simulink model "bumpem_control_system"  (R2021b)
settings: Solver=ode4  StartTime=0.0  StopTime=Inf  FixedStep=0.001  RelTol=1e-3
PostLoadFcn:
  | , if any(exist('dsrtsu_mdlpostloadfcn', 'file') == [2, 3, 6]), try dsrtsu_mdlpostloadfcn('Execute', bdroot); catch fprintf('Error in PostLoadFcn (dsrtsu_mdlpostloadfcn) for model "%s":\n %s\n', bdroot, lasterr); end, end,
libraries: rti1202lib_dac_class1 x4, simulink x4, dsparch4 x2, rti1202lib_adc_class1 x2
(part 1 of 2)
PreSaveFcn:
  | , if any(exist('dsmpb_private', 'file') == [2, 3, 6]), try, dsmpb_private('dsmpb_mdlclblib', 'PreSave', bdroot); catch, disp(lasterr); end, end,
CloseFcn:
  | , if any(exist('dsmpb_private', 'file') == [2, 3, 6]), try, dsmpb_private('dsmpb_mdlclblib', 'Close', bdroot); catch, disp(lasterr); end, end,
Description:
  | Standard RTI1202 template.
  | Supported MATLAB version:  R2018a.
settings Model: Tag=RTI1202  DSRTSU_INTERNAL_RTI_VER=520  DSRTSU_INTERNAL_RTI_TYPE=rti1202  RTICANMMDATA=struct('GeneralSetupData',struct('modelroot',['C:\Users\HuMoTech\Documents\Bump Em\simulink'],'generalsettings',struct('filesettings',struct('destfolder',struct('Name','RTICANMM_FILES','Check',1),'buildfolder',struct('Name','.','Check',1),'AbsDestfolder',struct('Name',['C:\Users\HuMoTech\Documents\Bump Em\simulink\RTICANMM_FILES']),'AbsBuildfolder',struct('Name',['C:\Users\HuMoTech\Documents\Bump Em\simulink']))),'options',struct('addpaths',1,'rmpaths',1,'addtrcexclusion',logical(1),'cannavigator',struct('checkmonitoring',0),'show_usrtrc',0,'use_usrtrc',0),'advanced',struct('options',[1 1 1 1 1 1 1 1 1 1 1 1 1 1 1 1 1 1 1 1 1 1 1 1 1 1 1 1 1 1 1 1 1 1 1 1 1 1 1 1 1 1 1 1 1 1 1 1 1 1 1 1 1 1 1 1 1 1 1 1 1 1 1 1 1 1 1 1 1 1 1 1 1 1 1 1 1 1 1 1 1 1 1 1 1 1 1 1 1 1 1 1 1 1 1 1 1 1 1 1]),'MPSetup',{{}},'modelname','latest_version_control_system_v2','block','latest_version_control_system_v2'))  DSRTSU_INTERNAL_RTIFLEXRAYCONFIG=110  DSRTSU_INTERNAL_RTIFPGA=110  DSMPB_DATASERVER_ModelPortLibVersion1=8  DSMPB_DATASERVER_DataServerVersion1=6  DSMPB_DATASERVER_DataServerStreamVersion1=3  Creator=HuMoTech  LastModifiedBy=maxia
settings SolverCC: AlgebraicLoopSolver=TrustRegion
settings DataIOCC: ReturnWorkspaceOutputs=off
settings OptimizationCC: BlockReduction=off  OptimizeBlockIOStorage=off  BufferReuse=off  GlobalBufferReuse=off  ExpressionFolding=off  LocalBlockOutputs=off  OptimizeDataStoreBuffers=off  BusAssignmentInplaceUpdate=off
settings DebuggingCC: SFMachineParentedDataDiag=warning  ArithmeticOperatorsInVariantConditions=warning
settings HardwareCC: ProdBitPerPointer=32  ProdBitPerSizeT=32  ProdBitPerPtrDiffT=32  ProdLargestAtomicInteger=Integer  ProdEndianess=BigEndian  ProdWordSize=32  ProdHWDeviceType=Custom Processor->Custom  TargetIntDivRoundTo=Zero  TargetEndianess=BigEndian  TargetHWDeviceType=Custom Processor->Custom
settings SFSimCC: SimUseLocalCustomCode=off  MATLABDynamicMemAlloc=off  CustomCodeUndefinedFunction=UseInterfaceOnly
settings RTWCC: Description=dSPACE DS1202 Hardware Platform  SystemTargetFile=rti1202.tlc  MakeCommand=make_rti  TemplateMakefile=rti1202.tmf  RTWUseLocalCustomCode=off
settings CodeAppCC: StateflowObjectComments=on
settings STFCustomTargetCC: ParMdlRefBuildCompliant=on  GRTInterface=off  SystemTargetFile=rti1202.tlc
settings GRTTargetCC: TargetLangStandard=C89/C90 (ANSI)  CompOptLevelCompliant=off  ConcurrentExecutionCompliant=off  CombineOutputUpdateFcns=off  MatFileLogging=off  CPPClassGenCompliant=off  UseToolchainInfoCompliant=off
settings ConfigComp: CovMetricSettings=dswe

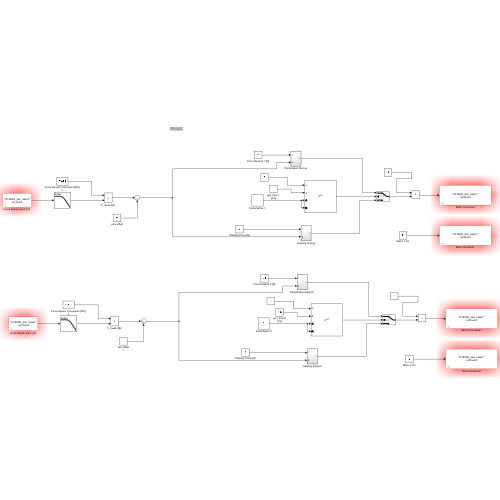
[thumbnail: Simulink's stored preview of the top-level diagram]
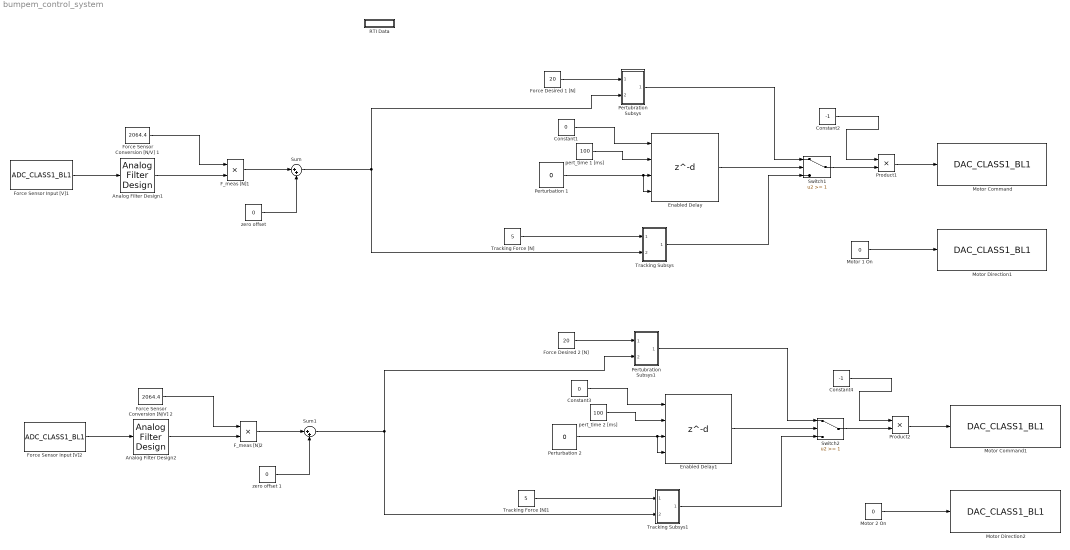
== system bumpem_control_system ==
  Analog Filter Design1 : dsparch4/Analog Filter Design  method=Butterworth  filttype=Lowpass  N=2  Wlo=40  Whi=80  Rp=2  Rs=40
  Analog Filter Design2 : dsparch4/Analog Filter Design  method=Butterworth  filttype=Lowpass  N=2  Wlo=40  Whi=80  Rp=2  Rs=40
  Constant1 : Constant  Value=0
  Constant2 : Constant  Value=-1
  Constant3 : Constant  Value=0
  Constant4 : Constant  Value=-1
  Enabled Delay : Delay  DelayLengthSource=Input port  DelayLength=300  DelayLengthUpperLimit=500  InitialCondition=1  ExternalReset=Either  ShowEnablePort=on
      settings: InputPortMap=u0,p1,e6,r5
  Enabled Delay1 : Delay  DelayLengthSource=Input port  DelayLength=300  DelayLengthUpperLimit=500  InitialCondition=1  ExternalReset=Either  ShowEnablePort=on
      settings: InputPortMap=u0,p1,e6,r5
  F_meas [N]1 : Product
  F_meas [N]2 : Product
  Force Desired 1 [N] : Constant  Value=20
  "Force Desired 2 [N] " : Constant  Value=20
  Force Sensor Conversion [N/V] 1 : Constant  Value=2064.4
  Force Sensor Conversion [N/V] 2 : Constant  Value=2064.4
  Force Sensor Input [V]1 : rti1202lib_adc_class1/ADC_CLASS1_BL1  DSProperties=struct('RTI',struct('Version',uint32(1),'BlockType',struct('isSLSource',uint8(1),'isSLSink',uint8(1),'isHWSource',uint8(0),'isHWSink',uint8(1),'isSetup',uint8(0),'isInline',uint8(1),'isNonInline',uint8(0),'isInterrupt',uint8(0),'isChannelwise',uint8(1)),'IOBoardType',{{'DS120X','STD','ADCC1'}},'UnitType','ADC','Identifier','ADC','DialogType','ML','BlockSet','NONE','SlaveProcessor','NONE'))  RTIBlockInterface=struct('InputPortsActive',0,'InputPortsWidth',int32(1),'InputPortsDataType',{{'SS_BOOLEAN'}},'InputPortsName',{{'Continue'}},'OutputPortsActive',[1 0],'OutputPortsWidth',int32([1 1]),'OutputPortsDataType',{{'SS_DOUBLE','SS_INT16'}},'OutputPortsName',{{'ADC','Status'}},'DialogFcn','rti120xstdadcc1adcgui','SampleTime',{{-1}},'InitLevel',3,'IconTransparency','on','BlockDisplay',{{['ADC CL1\nChannel: 1'],'center'}},'BlockName',struct('Token',{{'ADC_CLASS1_BL1'}}))  RTIBlockParameters=struct('ReadMode',{{1,'OFF',[1 2]}},'ChannelNo',{{1,'OFF',[]}},'ConversionMode',{{1,'OFF',[1 2]}},'TriggerSource',{{1,'OFF',[1 2]}},'TriggerLineIn',{{1,'OFF',[1 16]}},'SampleMode',{{1,'OFF',[1 2]}},'BurstTriggerSource',{{1,'OFF',[1 2]}},'BurstTriggerLine',{{1,'OFF',[1 16]}},'ConvTriggerSource',{{3,'OFF',[1 3]}},'ConvTriggerLine',{{1,'OFF',[1 16]}},'ConvPeriod',{{'100e-6','OFF',[1e-6 1.34]}},'ConvPeriodCheck',{{0,'OFF',[]}},'BurstSize',{{'10','OFF',[]}},'BurstSizeCheck',{{0,'OFF',[]}},'DataSetOffset',{{'0','OFF',[]}},'DataSetOffsetCheck',{{0,'OFF',[]}},'DataSetLength',{{'1','OFF',[]}},'DataSetLengthCheck',{{0,'OFF',[]}},'EnableTriggerEvent',{{0,'OFF',[0 1]}},'TriggerMode',{{2,'OFF',[1 3]}},'TriggerLineOut',{{1,'OFF',[1 16]}},'ADCSWStartEnable',{{0,'OFF',[0 1]}},'SampleTime',{{'-1','OFF',[-1 inf]}},'SampleTimeCheck',{{1,'OFF',[]}},'StatusPortEnable',{{0,'OFF',[0 1]}},'TLCFileName',{{'rti120xadc_c1_adc','OFF',[]}})  RTISFcnParameters=struct('ReadMode','int16','ChannelNo','int16','ConversionMode','int16','TriggerSource','int16','TriggerLineIn','int16','SampleMode','int16','BurstTriggerSource','int16','BurstTriggerLine','int16','ConvTriggerSource','int16','ConvTriggerLine','int16','ConvPeriod','double','BurstSize','int16','DataSetOffset','int16','DataSetLength','int16','EnableTriggerEvent','int16','TriggerMode','int16','TriggerLineOut','int16','ADCSWStartEnable','int16','SampleTime','double','StatusPortEnable','int16','TLCFileName','char')  RTIBlockParaDefault=struct('ReadMode',1,'ChannelNo',1,'ConversionMode',1,'TriggerSource',1,'TriggerLineIn',1,'SampleMode',1,'BurstTriggerSource',1,'BurstTriggerLine',1,'ConvTriggerSource',3,'ConvTriggerLine',1,'ConvPeriod',0.0001,'ConvPeriodCheck',0,'BurstSize',10,'BurstSizeCheck',0,'DataSetOffset',0,'DataSetOffsetCheck',0,'DataSetLength',1,'DataSetLengthCheck',0,'EnableTriggerEvent',0,'TriggerMode',2,'TriggerLineOut',1,'ADCSWStartEnable',0,'SampleTime',-1,'SampleTimeCheck',1,'StatusPortEnable',0,'TLCFileName','rti120xadc_c1_adc')
  Force Sensor Input [V]2 : rti1202lib_adc_class1/ADC_CLASS1_BL1  DSProperties=struct('RTI',struct('Version',uint32(1),'BlockType',struct('isSLSource',uint8(1),'isSLSink',uint8(1),'isHWSource',uint8(0),'isHWSink',uint8(1),'isSetup',uint8(0),'isInline',uint8(1),'isNonInline',uint8(0),'isInterrupt',uint8(0),'isChannelwise',uint8(1)),'IOBoardType',{{'DS120X','STD','ADCC1'}},'UnitType','ADC','Identifier','ADC','DialogType','ML','BlockSet','NONE','SlaveProcessor','NONE'))  RTIBlockInterface=struct('InputPortsActive',0,'InputPortsWidth',int32(1),'InputPortsDataType',{{'SS_BOOLEAN'}},'InputPortsName',{{'Continue'}},'OutputPortsActive',[1 0],'OutputPortsWidth',int32([1 1]),'OutputPortsDataType',{{'SS_DOUBLE','SS_INT16'}},'OutputPortsName',{{'ADC','Status'}},'DialogFcn','rti120xstdadcc1adcgui','SampleTime',{{-1}},'InitLevel',3,'IconTransparency','on','BlockDisplay',{{['ADC CL1\nChannel: 3'],'center'}},'BlockName',struct('Token',{{'ADC_CLASS1_BL1'}}))  RTIBlockParameters=struct('ReadMode',{{1,'OFF',[1 2]}},'ChannelNo',{{3,'OFF',[]}},'ConversionMode',{{1,'OFF',[1 2]}},'TriggerSource',{{1,'OFF',[1 2]}},'TriggerLineIn',{{1,'OFF',[1 16]}},'SampleMode',{{1,'OFF',[1 2]}},'BurstTriggerSource',{{1,'OFF',[1 2]}},'BurstTriggerLine',{{1,'OFF',[1 16]}},'ConvTriggerSource',{{3,'OFF',[1 3]}},'ConvTriggerLine',{{1,'OFF',[1 16]}},'ConvPeriod',{{'100e-6','OFF',[1e-6 1.34]}},'ConvPeriodCheck',{{0,'OFF',[]}},'BurstSize',{{'10','OFF',[]}},'BurstSizeCheck',{{0,'OFF',[]}},'DataSetOffset',{{'0','OFF',[]}},'DataSetOffsetCheck',{{0,'OFF',[]}},'DataSetLength',{{'1','OFF',[]}},'DataSetLengthCheck',{{0,'OFF',[]}},'EnableTriggerEvent',{{0,'OFF',[0 1]}},'TriggerMode',{{2,'OFF',[1 3]}},'TriggerLineOut',{{1,'OFF',[1 16]}},'ADCSWStartEnable',{{0,'OFF',[0 1]}},'SampleTime',{{'-1','OFF',[-1 inf]}},'SampleTimeCheck',{{1,'OFF',[]}},'StatusPortEnable',{{0,'OFF',[0 1]}},'TLCFileName',{{'rti120xadc_c1_adc','OFF',[]}})  RTISFcnParameters=struct('ReadMode','int16','ChannelNo','int16','ConversionMode','int16','TriggerSource','int16','TriggerLineIn','int16','SampleMode','int16','BurstTriggerSource','int16','BurstTriggerLine','int16','ConvTriggerSource','int16','ConvTriggerLine','int16','ConvPeriod','double','BurstSize','int16','DataSetOffset','int16','DataSetLength','int16','EnableTriggerEvent','int16','TriggerMode','int16','TriggerLineOut','int16','ADCSWStartEnable','int16','SampleTime','double','StatusPortEnable','int16','TLCFileName','char')  RTIBlockParaDefault=struct('ReadMode',1,'ChannelNo',1,'ConversionMode',1,'TriggerSource',1,'TriggerLineIn',1,'SampleMode',1,'BurstTriggerSource',1,'BurstTriggerLine',1,'ConvTriggerSource',3,'ConvTriggerLine',1,'ConvPeriod',0.0001,'ConvPeriodCheck',0,'BurstSize',10,'BurstSizeCheck',0,'DataSetOffset',0,'DataSetOffsetCheck',0,'DataSetLength',1,'DataSetLengthCheck',0,'EnableTriggerEvent',0,'TriggerMode',2,'TriggerLineOut',1,'ADCSWStartEnable',0,'SampleTime',-1,'SampleTimeCheck',1,'StatusPortEnable',0,'TLCFileName','rti120xadc_c1_adc')
  "Motor 1 On " : Constant  Value=0
  "Motor 2 On " : Constant  Value=0
  Motor Command : rti1202lib_dac_class1/DAC_CLASS1_BL1  DSProperties=struct('RTI',struct('Version',uint32(2),'BlockType',struct('isSLSource',uint8(0),'isSLSink',uint8(1),'isHWSource',uint8(0),'isHWSink',uint8(1),'isSetup',uint8(0),'isInline',uint8(1),'isNonInline',uint8(0),'isInterrupt',uint8(0),'isChannelwise',uint8(1)),'IOBoardType',{{'DS120X','STD','DACC1'}},'UnitType','DAC','Identifier','DAC','DialogType','ML','BlockSet','NONE','SlaveProcessor','NONE'))  RTIBlockInterface=struct('InputPortsActive',1,'InputPortsWidth',int32(1),'InputPortsDataType',{{'SS_DOUBLE'}},'InputPortsName',{{['DAC 1']}},'DialogFcn','rti120xstddacc1dacgui','InitLevel',3,'IconTransparency','on','BlockDisplay',{{['DAC CL1\nChannel: 1'],'center'}},'BlockName',struct('Token',{{'DAC_CLASS1_BL1'}}))  RTIBlockParameters=struct('ChannelNo',{{1,'OFF',[]}},'ChannelNumOf',{{1,'OFF',[]}},'InitialValue1',{{0,'OFF',[-10 10]}},'InitialValue2',{{0,'OFF',[-10 10]}},'InitialValue3',{{0,'OFF',[-10 10]}},'InitialValue4',{{0,'OFF',[-10 10]}},'InitialValue5',{{0,'OFF',[-10 10]}},'InitialValue6',{{0,'OFF',[-10 10]}},'InitialValue7',{{0,'OFF',[-10 10]}},'InitialValue8',{{0,'OFF',[-10 10]}},'InitialValue9',{{0,'OFF',[-10 10]}},'InitialValue10',{{0,'OFF',[-10 10]}},'InitialValue11',{{0,'OFF',[-10 10]}},'InitialValue12',{{0,'OFF',[-10 10]}},'InitialValue13',{{0,'OFF',[-10 10]}},'InitialValue14',{{0,'OFF',[-10 10]}},'InitialValue15',{{0,'OFF',[-10 10]}},'InitialValue16',{{0,'OFF',[-10 10]}},'OutputMode',{{ones(1,16),'OFF',[1 2]}},'TermValue1',{{0,'OFF',[-10 10]}},'TermValue2',{{0,'OFF',[-10 10]}},'TermValue3',{{0,'OFF',[-10 10]}},'TermValue4',{{0,'OFF',[-10 10]}},'TermValue5',{{0,'OFF',[-10 10]}},'TermValue6',{{0,'OFF',[-10 10]}},'TermValue7',{{0,'OFF',[-10 10]}},'TermValue8',{{0,'OFF',[-10 10]}},'TermValue9',{{0,'OFF',[-10 10]}},'TermValue10',{{0,'OFF',[-10 10]}},'TermValue11',{{0,'OFF',[-10 10]}},'TermValue12',{{0,'OFF',[-10 10]}},'TermValue13',{{0,'OFF',[-10 10]}},'TermValue14',{{0,'OFF',[-10 10]}},'TermValue15',{{0,'OFF',[-10 10]}},'TermValue16',{{0,'OFF',[-10 10]}},'EnableTermMode',{{0,'OFF',[0 1]}},'TLCFileName',{{'rti120xdac_c1_dac','OFF',[]}},'InitialValueBuildCheck1',{{0,'OFF',[]}},'InitialValueBuildCheck2',{{0,'OFF',[]}},'InitialValueBuildCheck3',{{0,'OFF',[]}},'InitialValueBuildCheck4',{{0,'OFF',[]}},'InitialValueBuildCheck5',{{0,'OFF',[]}},'InitialValueBuildCheck6',{{0,'OFF',[]}},'InitialValueBuildCheck7',{{0,'OFF',[]}},'InitialValueBuildCheck8',{{0,'OFF',[]}},'InitialValueBuildCheck9',{{0,'OFF',[]}},'InitialValueBuildCheck10',{{0,'OFF',[]}},'InitialValueBuildCheck11',{{0,'OFF',[]}},'InitialValueBuildCheck12',{{0,'OFF',[]}},'InitialValueBuildCheck13',{{0,'OFF',[]}},'InitialValueBuildCheck14',{{0,'OFF',[]}},'InitialValueBuildCheck15',{{0,'OFF',[]}},'InitialValueBuildCheck16',{{0,'OFF',[]}},'TermValueBuildCheck1',{{0,'OFF',[]}},'TermValueBuildCheck2',{{0,'OFF',[]}},'TermValueBuildCheck3',{{0,'OFF',[]}},'TermValueBuildCheck4',{{0,'OFF',[]}},'TermValueBuildCheck5',{{0,'OFF',[]}},'TermValueBuildCheck6',{{0,'OFF',[]}},'TermValueBuildCheck7',{{0,'OFF',[]}},'TermValueBuildCheck8',{{0,'OFF',[]}},'TermValueBuildCheck9',{{0,'OFF',[]}},'TermValueBuildCheck10',{{0,'OFF',[]}},'TermValueBuildCheck11',{{0,'OFF',[]}},'TermValueBuildCheck12',{{0,'OFF',[]}},'TermValueBuildCheck13',{{0,'OFF',[]}},'TermValueBuildCheck14',{{0,'OFF',[]}},'TermValueBuildCheck15',{{0,'OFF',[]}},'TermValueBuildCheck16',{{0,'OFF',[]}})  RTISFcnParameters=struct('ChannelNo','int16','ChannelNumOf','int16','InitialValue1','double','InitialValue2','double','InitialValue3','double','InitialValue4','double','InitialValue5','double','InitialValue6','double','InitialValue7','double','InitialValue8','double','InitialValue9','double','InitialValue10','double','InitialValue11','double','InitialValue12','double','InitialValue13','double','InitialValue14','double','InitialValue15','double','InitialValue16','double','OutputMode','int16','TermValue1','double','TermValue2','double','TermValue3','double','TermValue4','double','TermValue5','double','TermValue6','double','TermValue7','double','TermValue8','double','TermValue9','double','TermValue10','double','TermValue11','double','TermValue12','double','TermValue13','double','TermValue14','double','TermValue15','double','TermValue16','double','EnableTermMode','int16','TLCFileName','char')  RTIBlockParaDefault=struct('ChannelNo',1,'ChannelNumOf',1,'InitialValue1',0,'InitialValue2',0,'InitialValue3',0,'InitialValue4',0,'InitialValue5',0,'InitialValue6',0,'InitialValue7',0,'InitialValue8',0,'InitialValue9',0,'InitialValue10',0,'InitialValue11',0,'InitialValue12',0,'InitialValue13',0,'InitialValue14',0,'InitialValue15',0,'InitialValue16',0,'OutputMode',ones(1,16),'TermValue1',0,'TermValue2',0,'TermValue3',0,'TermValue4',0,'TermValue5',0,'TermValue6',0,'TermValue7',0,'TermValue8',0,'TermValue9',0,'TermValue10',0,'TermValue11',0,'TermValue12',0,'TermValue13',0,'TermValue14',0,'TermValue15',0,'TermValue16',0,'EnableTermMode',0,'TLCFileName','rti120xdac_c1_dac','InitialValueBuildCheck1',0,'InitialValueBuildCheck2',0,'InitialValueBuildCheck3',0,'InitialValueBuildCheck4',0,'InitialValueBuildCheck5',0,'InitialValueBuildCheck6',0,'InitialValueBuildCheck7',0,'InitialValueBuildCheck8',0,'InitialValueBuildCheck9',0,'InitialValueBuildCheck10',0,'InitialValueBuildCheck11',0,'InitialValueBuildCheck12',0,'InitialValueBuildCheck13',0,'InitialValueBuildCheck14',0,'InitialValueBuildCheck15',0,'InitialValueBuildCheck16',0,'TermValueBuildCheck1',0,'TermValueBuildCheck2',0,'TermValueBuildCheck3',0,'TermValueBuildCheck4',0,'TermValueBuildCheck5',0,'TermValueBuildCheck6',0,'TermValueBuildCheck7',0,'TermValueBuildCheck8',0,'TermValueBuildCheck9',0,'TermValueBuildCheck10',0,'TermValueBuildCheck11',0,'TermValueBuildCheck12',0,'TermValueBuildCheck13',0,'TermValueBuildCheck14',0,'TermValueBuildCheck15',0,'TermValueBuildCheck16',0)
  Motor Command1 : rti1202lib_dac_class1/DAC_CLASS1_BL1  DSProperties=struct('RTI',struct('Version',uint32(2),'BlockType',struct('isSLSource',uint8(0),'isSLSink',uint8(1),'isHWSource',uint8(0),'isHWSink',uint8(1),'isSetup',uint8(0),'isInline',uint8(1),'isNonInline',uint8(0),'isInterrupt',uint8(0),'isChannelwise',uint8(1)),'IOBoardType',{{'DS120X','STD','DACC1'}},'UnitType','DAC','Identifier','DAC','DialogType','ML','BlockSet','NONE','SlaveProcessor','NONE'))  RTIBlockInterface=struct('InputPortsActive',1,'InputPortsWidth',int32(1),'InputPortsDataType',{{'SS_DOUBLE'}},'InputPortsName',{{['DAC 3']}},'DialogFcn','rti120xstddacc1dacgui','InitLevel',3,'IconTransparency','on','BlockDisplay',{{['DAC CL1\nChannel: 3'],'center'}},'BlockName',struct('Token',{{'DAC_CLASS1_BL1'}}))  RTIBlockParameters=struct('ChannelNo',{{3,'OFF',[]}},'ChannelNumOf',{{1,'OFF',[]}},'InitialValue1',{{'0','OFF',[-10 10]}},'InitialValue2',{{'0','OFF',[-10 10]}},'InitialValue3',{{'0','OFF',[-10 10]}},'InitialValue4',{{'0','OFF',[-10 10]}},'InitialValue5',{{'0','OFF',[-10 10]}},'InitialValue6',{{'0','OFF',[-10 10]}},'InitialValue7',{{'0','OFF',[-10 10]}},'InitialValue8',{{'0','OFF',[-10 10]}},'InitialValue9',{{'0','OFF',[-10 10]}},'InitialValue10',{{'0','OFF',[-10 10]}},'InitialValue11',{{'0','OFF',[-10 10]}},'InitialValue12',{{'0','OFF',[-10 10]}},'InitialValue13',{{'0','OFF',[-10 10]}},'InitialValue14',{{'0','OFF',[-10 10]}},'InitialValue15',{{'0','OFF',[-10 10]}},'InitialValue16',{{'0','OFF',[-10 10]}},'OutputMode',{{ones(1,16),'OFF',[1 2]}},'TermValue1',{{'0','OFF',[-10 10]}},'TermValue2',{{'0','OFF',[-10 10]}},'TermValue3',{{'0','OFF',[-10 10]}},'TermValue4',{{'0','OFF',[-10 10]}},'TermValue5',{{'0','OFF',[-10 10]}},'TermValue6',{{'0','OFF',[-10 10]}},'TermValue7',{{'0','OFF',[-10 10]}},'TermValue8',{{'0','OFF',[-10 10]}},'TermValue9',{{'0','OFF',[-10 10]}},'TermValue10',{{'0','OFF',[-10 10]}},'TermValue11',{{'0','OFF',[-10 10]}},'TermValue12',{{'0','OFF',[-10 10]}},'TermValue13',{{'0','OFF',[-10 10]}},'TermValue14',{{'0','OFF',[-10 10]}},'TermValue15',{{'0','OFF',[-10 10]}},'TermValue16',{{'0','OFF',[-10 10]}},'EnableTermMode',{{0,'OFF',[0 1]}},'TLCFileName',{{'rti120xdac_c1_dac','OFF',[]}},'InitialValueBuildCheck1',{{0,'OFF',[]}},'InitialValueBuildCheck2',{{0,'OFF',[]}},'InitialValueBuildCheck3',{{1,'OFF',[]}},'InitialValueBuildCheck4',{{0,'OFF',[]}},'InitialValueBuildCheck5',{{0,'OFF',[]}},'InitialValueBuildCheck6',{{0,'OFF',[]}},'InitialValueBuildCheck7',{{0,'OFF',[]}},'InitialValueBuildCheck8',{{0,'OFF',[]}},'InitialValueBuildCheck9',{{0,'OFF',[]}},'InitialValueBuildCheck10',{{0,'OFF',[]}},'InitialValueBuildCheck11',{{0,'OFF',[]}},'InitialValueBuildCheck12',{{0,'OFF',[]}},'InitialValueBuildCheck13',{{0,'OFF',[]}},'InitialValueBuildCheck14',{{0,'OFF',[]}},'InitialValueBuildCheck15',{{0,'OFF',[]}},'InitialValueBuildCheck16',{{0,'OFF',[]}},'TermValueBuildCheck1',{{0,'OFF',[]}},'TermValueBuildCheck2',{{0,'OFF',[]}},'TermValueBuildCheck3',{{0,'OFF',[]}},'TermValueBuildCheck4',{{0,'OFF',[]}},'TermValueBuildCheck5',{{0,'OFF',[]}},'TermValueBuildCheck6',{{0,'OFF',[]}},'TermValueBuildCheck7',{{0,'OFF',[]}},'TermValueBuildCheck8',{{0,'OFF',[]}},'TermValueBuildCheck9',{{0,'OFF',[]}},'TermValueBuildCheck10',{{0,'OFF',[]}},'TermValueBuildCheck11',{{0,'OFF',[]}},'TermValueBuildCheck12',{{0,'OFF',[]}},'TermValueBuildCheck13',{{0,'OFF',[]}},'TermValueBuildCheck14',{{0,'OFF',[]}},'TermValueBuildCheck15',{{0,'OFF',[]}},'TermValueBuildCheck16',{{0,'OFF',[]}})  RTISFcnParameters=struct('ChannelNo','int16','ChannelNumOf','int16','InitialValue1','double','InitialValue2','double','InitialValue3','double','InitialValue4','double','InitialValue5','double','InitialValue6','double','InitialValue7','double','InitialValue8','double','InitialValue9','double','InitialValue10','double','InitialValue11','double','InitialValue12','double','InitialValue13','double','InitialValue14','double','InitialValue15','double','InitialValue16','double','OutputMode','int16','TermValue1','double','TermValue2','double','TermValue3','double','TermValue4','double','TermValue5','double','TermValue6','double','TermValue7','double','TermValue8','double','TermValue9','double','TermValue10','double','TermValue11','double','TermValue12','double','TermValue13','double','TermValue14','double','TermValue15','double','TermValue16','double','EnableTermMode','int16','TLCFileName','char')  RTIBlockParaDefault=struct('ChannelNo',1,'ChannelNumOf',1,'InitialValue1',0,'InitialValue2',0,'InitialValue3',0,'InitialValue4',0,'InitialValue5',0,'InitialValue6',0,'InitialValue7',0,'InitialValue8',0,'InitialValue9',0,'InitialValue10',0,'InitialValue11',0,'InitialValue12',0,'InitialValue13',0,'InitialValue14',0,'InitialValue15',0,'InitialValue16',0,'OutputMode',ones(1,16),'TermValue1',0,'TermValue2',0,'TermValue3',0,'TermValue4',0,'TermValue5',0,'TermValue6',0,'TermValue7',0,'TermValue8',0,'TermValue9',0,'TermValue10',0,'TermValue11',0,'TermValue12',0,'TermValue13',0,'TermValue14',0,'TermValue15',0,'TermValue16',0,'EnableTermMode',0,'TLCFileName','rti120xdac_c1_dac','InitialValueBuildCheck1',0,'InitialValueBuildCheck2',0,'InitialValueBuildCheck3',0,'InitialValueBuildCheck4',0,'InitialValueBuildCheck5',0,'InitialValueBuildCheck6',0,'InitialValueBuildCheck7',0,'InitialValueBuildCheck8',0,'InitialValueBuildCheck9',0,'InitialValueBuildCheck10',0,'InitialValueBuildCheck11',0,'InitialValueBuildCheck12',0,'InitialValueBuildCheck13',0,'InitialValueBuildCheck14',0,'InitialValueBuildCheck15',0,'InitialValueBuildCheck16',0,'TermValueBuildCheck1',0,'TermValueBuildCheck2',0,'TermValueBuildCheck3',0,'TermValueBuildCheck4',0,'TermValueBuildCheck5',0,'TermValueBuildCheck6',0,'TermValueBuildCheck7',0,'TermValueBuildCheck8',0,'TermValueBuildCheck9',0,'TermValueBuildCheck10',0,'TermValueBuildCheck11',0,'TermValueBuildCheck12',0,'TermValueBuildCheck13',0,'TermValueBuildCheck14',0,'TermValueBuildCheck15',0,'TermValueBuildCheck16',0)
  Motor Direction1 : rti1202lib_dac_class1/DAC_CLASS1_BL1  DSProperties=struct('RTI',struct('Version',uint32(2),'BlockType',struct('isSLSource',uint8(0),'isSLSink',uint8(1),'isHWSource',uint8(0),'isHWSink',uint8(1),'isSetup',uint8(0),'isInline',uint8(1),'isNonInline',uint8(0),'isInterrupt',uint8(0),'isChannelwise',uint8(1)),'IOBoardType',{{'DS120X','STD','DACC1'}},'UnitType','DAC','Identifier','DAC','DialogType','ML','BlockSet','NONE','SlaveProcessor','NONE'))  RTIBlockInterface=struct('InputPortsActive',1,'InputPortsWidth',int32(1),'InputPortsDataType',{{'SS_DOUBLE'}},'InputPortsName',{{['DAC 2']}},'DialogFcn','rti120xstddacc1dacgui','InitLevel',3,'IconTransparency','on','BlockDisplay',{{['DAC CL1\nChannel: 2'],'center'}},'BlockName',struct('Token',{{'DAC_CLASS1_BL1'}}))  RTIBlockParameters=struct('ChannelNo',{{2,'OFF',[]}},'ChannelNumOf',{{1,'OFF',[]}},'InitialValue1',{{'0','OFF',[-10 10]}},'InitialValue2',{{'0','OFF',[-10 10]}},'InitialValue3',{{'0','OFF',[-10 10]}},'InitialValue4',{{'0','OFF',[-10 10]}},'InitialValue5',{{'0','OFF',[-10 10]}},'InitialValue6',{{'0','OFF',[-10 10]}},'InitialValue7',{{'0','OFF',[-10 10]}},'InitialValue8',{{'0','OFF',[-10 10]}},'InitialValue9',{{'0','OFF',[-10 10]}},'InitialValue10',{{'0','OFF',[-10 10]}},'InitialValue11',{{'0','OFF',[-10 10]}},'InitialValue12',{{'0','OFF',[-10 10]}},'InitialValue13',{{'0','OFF',[-10 10]}},'InitialValue14',{{'0','OFF',[-10 10]}},'InitialValue15',{{'0','OFF',[-10 10]}},'InitialValue16',{{'0','OFF',[-10 10]}},'OutputMode',{{ones(1,16),'OFF',[1 2]}},'TermValue1',{{'0','OFF',[-10 10]}},'TermValue2',{{'0','OFF',[-10 10]}},'TermValue3',{{'0','OFF',[-10 10]}},'TermValue4',{{'0','OFF',[-10 10]}},'TermValue5',{{'0','OFF',[-10 10]}},'TermValue6',{{'0','OFF',[-10 10]}},'TermValue7',{{'0','OFF',[-10 10]}},'TermValue8',{{'0','OFF',[-10 10]}},'TermValue9',{{'0','OFF',[-10 10]}},'TermValue10',{{'0','OFF',[-10 10]}},'TermValue11',{{'0','OFF',[-10 10]}},'TermValue12',{{'0','OFF',[-10 10]}},'TermValue13',{{'0','OFF',[-10 10]}},'TermValue14',{{'0','OFF',[-10 10]}},'TermValue15',{{'0','OFF',[-10 10]}},'TermValue16',{{'0','OFF',[-10 10]}},'EnableTermMode',{{0,'OFF',[0 1]}},'TLCFileName',{{'rti120xdac_c1_dac','OFF',[]}},'InitialValueBuildCheck1',{{0,'OFF',[]}},'InitialValueBuildCheck2',{{1,'OFF',[]}},'InitialValueBuildCheck3',{{0,'OFF',[]}},'InitialValueBuildCheck4',{{0,'OFF',[]}},'InitialValueBuildCheck5',{{0,'OFF',[]}},'InitialValueBuildCheck6',{{0,'OFF',[]}},'InitialValueBuildCheck7',{{0,'OFF',[]}},'InitialValueBuildCheck8',{{0,'OFF',[]}},'InitialValueBuildCheck9',{{0,'OFF',[]}},'InitialValueBuildCheck10',{{0,'OFF',[]}},'InitialValueBuildCheck11',{{0,'OFF',[]}},'InitialValueBuildCheck12',{{0,'OFF',[]}},'InitialValueBuildCheck13',{{0,'OFF',[]}},'InitialValueBuildCheck14',{{0,'OFF',[]}},'InitialValueBuildCheck15',{{0,'OFF',[]}},'InitialValueBuildCheck16',{{0,'OFF',[]}},'TermValueBuildCheck1',{{0,'OFF',[]}},'TermValueBuildCheck2',{{0,'OFF',[]}},'TermValueBuildCheck3',{{0,'OFF',[]}},'TermValueBuildCheck4',{{0,'OFF',[]}},'TermValueBuildCheck5',{{0,'OFF',[]}},'TermValueBuildCheck6',{{0,'OFF',[]}},'TermValueBuildCheck7',{{0,'OFF',[]}},'TermValueBuildCheck8',{{0,'OFF',[]}},'TermValueBuildCheck9',{{0,'OFF',[]}},'TermValueBuildCheck10',{{0,'OFF',[]}},'TermValueBuildCheck11',{{0,'OFF',[]}},'TermValueBuildCheck12',{{0,'OFF',[]}},'TermValueBuildCheck13',{{0,'OFF',[]}},'TermValueBuildCheck14',{{0,'OFF',[]}},'TermValueBuildCheck15',{{0,'OFF',[]}},'TermValueBuildCheck16',{{0,'OFF',[]}})  RTISFcnParameters=struct('ChannelNo','int16','ChannelNumOf','int16','InitialValue1','double','InitialValue2','double','InitialValue3','double','InitialValue4','double','InitialValue5','double','InitialValue6','double','InitialValue7','double','InitialValue8','double','InitialValue9','double','InitialValue10','double','InitialValue11','double','InitialValue12','double','InitialValue13','double','InitialValue14','double','InitialValue15','double','InitialValue16','double','OutputMode','int16','TermValue1','double','TermValue2','double','TermValue3','double','TermValue4','double','TermValue5','double','TermValue6','double','TermValue7','double','TermValue8','double','TermValue9','double','TermValue10','double','TermValue11','double','TermValue12','double','TermValue13','double','TermValue14','double','TermValue15','double','TermValue16','double','EnableTermMode','int16','TLCFileName','char')  RTIBlockParaDefault=struct('ChannelNo',1,'ChannelNumOf',1,'InitialValue1',0,'InitialValue2',0,'InitialValue3',0,'InitialValue4',0,'InitialValue5',0,'InitialValue6',0,'InitialValue7',0,'InitialValue8',0,'InitialValue9',0,'InitialValue10',0,'InitialValue11',0,'InitialValue12',0,'InitialValue13',0,'InitialValue14',0,'InitialValue15',0,'InitialValue16',0,'OutputMode',ones(1,16),'TermValue1',0,'TermValue2',0,'TermValue3',0,'TermValue4',0,'TermValue5',0,'TermValue6',0,'TermValue7',0,'TermValue8',0,'TermValue9',0,'TermValue10',0,'TermValue11',0,'TermValue12',0,'TermValue13',0,'TermValue14',0,'TermValue15',0,'TermValue16',0,'EnableTermMode',0,'TLCFileName','rti120xdac_c1_dac','InitialValueBuildCheck1',0,'InitialValueBuildCheck2',0,'InitialValueBuildCheck3',0,'InitialValueBuildCheck4',0,'InitialValueBuildCheck5',0,'InitialValueBuildCheck6',0,'InitialValueBuildCheck7',0,'InitialValueBuildCheck8',0,'InitialValueBuildCheck9',0,'InitialValueBuildCheck10',0,'InitialValueBuildCheck11',0,'InitialValueBuildCheck12',0,'InitialValueBuildCheck13',0,'InitialValueBuildCheck14',0,'InitialValueBuildCheck15',0,'InitialValueBuildCheck16',0,'TermValueBuildCheck1',0,'TermValueBuildCheck2',0,'TermValueBuildCheck3',0,'TermValueBuildCheck4',0,'TermValueBuildCheck5',0,'TermValueBuildCheck6',0,'TermValueBuildCheck7',0,'TermValueBuildCheck8',0,'TermValueBuildCheck9',0,'TermValueBuildCheck10',0,'TermValueBuildCheck11',0,'TermValueBuildCheck12',0,'TermValueBuildCheck13',0,'TermValueBuildCheck14',0,'TermValueBuildCheck15',0,'TermValueBuildCheck16',0)
  Motor Direction2 : rti1202lib_dac_class1/DAC_CLASS1_BL1  DSProperties=struct('RTI',struct('Version',uint32(2),'BlockType',struct('isSLSource',uint8(0),'isSLSink',uint8(1),'isHWSource',uint8(0),'isHWSink',uint8(1),'isSetup',uint8(0),'isInline',uint8(1),'isNonInline',uint8(0),'isInterrupt',uint8(0),'isChannelwise',uint8(1)),'IOBoardType',{{'DS120X','STD','DACC1'}},'UnitType','DAC','Identifier','DAC','DialogType','ML','BlockSet','NONE','SlaveProcessor','NONE'))  RTIBlockInterface=struct('InputPortsActive',1,'InputPortsWidth',int32(1),'InputPortsDataType',{{'SS_DOUBLE'}},'InputPortsName',{{['DAC 4']}},'DialogFcn','rti120xstddacc1dacgui','InitLevel',3,'IconTransparency','on','BlockDisplay',{{['DAC CL1\nChannel: 4'],'center'}},'BlockName',struct('Token',{{'DAC_CLASS1_BL1'}}))  RTIBlockParameters=struct('ChannelNo',{{4,'OFF',[]}},'ChannelNumOf',{{1,'OFF',[]}},'InitialValue1',{{'0','OFF',[-10 10]}},'InitialValue2',{{'0','OFF',[-10 10]}},'InitialValue3',{{'0','OFF',[-10 10]}},'InitialValue4',{{'0','OFF',[-10 10]}},'InitialValue5',{{'0','OFF',[-10 10]}},'InitialValue6',{{'0','OFF',[-10 10]}},'InitialValue7',{{'0','OFF',[-10 10]}},'InitialValue8',{{'0','OFF',[-10 10]}},'InitialValue9',{{'0','OFF',[-10 10]}},'InitialValue10',{{'0','OFF',[-10 10]}},'InitialValue11',{{'0','OFF',[-10 10]}},'InitialValue12',{{'0','OFF',[-10 10]}},'InitialValue13',{{'0','OFF',[-10 10]}},'InitialValue14',{{'0','OFF',[-10 10]}},'InitialValue15',{{'0','OFF',[-10 10]}},'InitialValue16',{{'0','OFF',[-10 10]}},'OutputMode',{{ones(1,16),'OFF',[1 2]}},'TermValue1',{{'0','OFF',[-10 10]}},'TermValue2',{{'0','OFF',[-10 10]}},'TermValue3',{{'0','OFF',[-10 10]}},'TermValue4',{{'0','OFF',[-10 10]}},'TermValue5',{{'0','OFF',[-10 10]}},'TermValue6',{{'0','OFF',[-10 10]}},'TermValue7',{{'0','OFF',[-10 10]}},'TermValue8',{{'0','OFF',[-10 10]}},'TermValue9',{{'0','OFF',[-10 10]}},'TermValue10',{{'0','OFF',[-10 10]}},'TermValue11',{{'0','OFF',[-10 10]}},'TermValue12',{{'0','OFF',[-10 10]}},'TermValue13',{{'0','OFF',[-10 10]}},'TermValue14',{{'0','OFF',[-10 10]}},'TermValue15',{{'0','OFF',[-10 10]}},'TermValue16',{{'0','OFF',[-10 10]}},'EnableTermMode',{{0,'OFF',[0 1]}},'TLCFileName',{{'rti120xdac_c1_dac','OFF',[]}},'InitialValueBuildCheck1',{{0,'OFF',[]}},'InitialValueBuildCheck2',{{0,'OFF',[]}},'InitialValueBuildCheck3',{{0,'OFF',[]}},'InitialValueBuildCheck4',{{1,'OFF',[]}},'InitialValueBuildCheck5',{{0,'OFF',[]}},'InitialValueBuildCheck6',{{0,'OFF',[]}},'InitialValueBuildCheck7',{{0,'OFF',[]}},'InitialValueBuildCheck8',{{0,'OFF',[]}},'InitialValueBuildCheck9',{{0,'OFF',[]}},'InitialValueBuildCheck10',{{0,'OFF',[]}},'InitialValueBuildCheck11',{{0,'OFF',[]}},'InitialValueBuildCheck12',{{0,'OFF',[]}},'InitialValueBuildCheck13',{{0,'OFF',[]}},'InitialValueBuildCheck14',{{0,'OFF',[]}},'InitialValueBuildCheck15',{{0,'OFF',[]}},'InitialValueBuildCheck16',{{0,'OFF',[]}},'TermValueBuildCheck1',{{0,'OFF',[]}},'TermValueBuildCheck2',{{0,'OFF',[]}},'TermValueBuildCheck3',{{0,'OFF',[]}},'TermValueBuildCheck4',{{0,'OFF',[]}},'TermValueBuildCheck5',{{0,'OFF',[]}},'TermValueBuildCheck6',{{0,'OFF',[]}},'TermValueBuildCheck7',{{0,'OFF',[]}},'TermValueBuildCheck8',{{0,'OFF',[]}},'TermValueBuildCheck9',{{0,'OFF',[]}},'TermValueBuildCheck10',{{0,'OFF',[]}},'TermValueBuildCheck11',{{0,'OFF',[]}},'TermValueBuildCheck12',{{0,'OFF',[]}},'TermValueBuildCheck13',{{0,'OFF',[]}},'TermValueBuildCheck14',{{0,'OFF',[]}},'TermValueBuildCheck15',{{0,'OFF',[]}},'TermValueBuildCheck16',{{0,'OFF',[]}})  RTISFcnParameters=struct('ChannelNo','int16','ChannelNumOf','int16','InitialValue1','double','InitialValue2','double','InitialValue3','double','InitialValue4','double','InitialValue5','double','InitialValue6','double','InitialValue7','double','InitialValue8','double','InitialValue9','double','InitialValue10','double','InitialValue11','double','InitialValue12','double','InitialValue13','double','InitialValue14','double','InitialValue15','double','InitialValue16','double','OutputMode','int16','TermValue1','double','TermValue2','double','TermValue3','double','TermValue4','double','TermValue5','double','TermValue6','double','TermValue7','double','TermValue8','double','TermValue9','double','TermValue10','double','TermValue11','double','TermValue12','double','TermValue13','double','TermValue14','double','TermValue15','double','TermValue16','double','EnableTermMode','int16','TLCFileName','char')  RTIBlockParaDefault=struct('ChannelNo',1,'ChannelNumOf',1,'InitialValue1',0,'InitialValue2',0,'InitialValue3',0,'InitialValue4',0,'InitialValue5',0,'InitialValue6',0,'InitialValue7',0,'InitialValue8',0,'InitialValue9',0,'InitialValue10',0,'InitialValue11',0,'InitialValue12',0,'InitialValue13',0,'InitialValue14',0,'InitialValue15',0,'InitialValue16',0,'OutputMode',ones(1,16),'TermValue1',0,'TermValue2',0,'TermValue3',0,'TermValue4',0,'TermValue5',0,'TermValue6',0,'TermValue7',0,'TermValue8',0,'TermValue9',0,'TermValue10',0,'TermValue11',0,'TermValue12',0,'TermValue13',0,'TermValue14',0,'TermValue15',0,'TermValue16',0,'EnableTermMode',0,'TLCFileName','rti120xdac_c1_dac','InitialValueBuildCheck1',0,'InitialValueBuildCheck2',0,'InitialValueBuildCheck3',0,'InitialValueBuildCheck4',0,'InitialValueBuildCheck5',0,'InitialValueBuildCheck6',0,'InitialValueBuildCheck7',0,'InitialValueBuildCheck8',0,'InitialValueBuildCheck9',0,'InitialValueBuildCheck10',0,'InitialValueBuildCheck11',0,'InitialValueBuildCheck12',0,'InitialValueBuildCheck13',0,'InitialValueBuildCheck14',0,'InitialValueBuildCheck15',0,'InitialValueBuildCheck16',0,'TermValueBuildCheck1',0,'TermValueBuildCheck2',0,'TermValueBuildCheck3',0,'TermValueBuildCheck4',0,'TermValueBuildCheck5',0,'TermValueBuildCheck6',0,'TermValueBuildCheck7',0,'TermValueBuildCheck8',0,'TermValueBuildCheck9',0,'TermValueBuildCheck10',0,'TermValueBuildCheck11',0,'TermValueBuildCheck12',0,'TermValueBuildCheck13',0,'TermValueBuildCheck14',0,'TermValueBuildCheck15',0,'TermValueBuildCheck16',0)
  Pertubration Subsys : Subsystem
  Pertubration Subsys1 : Subsystem
  "Perturbation 1 " : Constant  Value=0
  Perturbation 2 : Constant  Value=0
  Product1 : Product
  Product2 : Product
  RTI Data : Subsystem  Tag=struct('RTIDataServer',struct('RTIDataServerVs','2','RTIModelDescription','struct(''main'',''latest_version_control_system_v2'',''sub'','''',''isMp'',0)'))  LoadFcn="if exist('rtidc'), try,  rtidc('DataHostBlockClbLoad', gcbh); catch, disp(['Warning: ''LoadFcn'' for RTI Data block failed: ' lasterr]); end, end,"  mask(RTI_DATA_HOST){}
      mask help:
      | RTI Data Block.
      | This block is used by RTI to store internal model-dependent data.
      | Please keep this block on the root level of the model. Deleting this block will result in data loss.
      |
      | NEVER DELETE OR COPY THIS BLOCK!
      settings: CopyFcn="if exist('rtidc'), try,  rtidc('DataHostBlockClbCopy', gcbh); catch, disp(['Warning: ''CopyFcn'' for RTI Data block failed: ' lasterr]); end, end,"  DeleteFcn="if exist('rtidc'), try,  rtidc('DataHostBlockClbDelete', gcbh); catch, disp(['Warning: ''DeleteFcn'' for RTI Data block failed: ' lasterr]); end, end,"  ModelCloseFcn="if exist('rtidc'), try,  rtidc('DataHostBlockClbModelClose', gcbh); catch, disp(['Warning: ''ModelCloseFcn'' for RTI Data block failed: ' lasterr]); end, end,"  PreSaveFcn="if exist('rtidc'), try,  rtidc('DataHostBlockClbPreSave', gcbh); catch, disp(['Warning: ''PreSaveFcn'' for RTI Data block failed: ' lasterr]); end, end,"  PostSaveFcn="if exist('rtidc'), try,  rtidc('DataHostBlockClbPostSave', gcbh); catch, disp(['Warning: ''PostSaveFcn'' for RTI Data block failed: ' lasterr]); end, end,"  NameChangeFcn="if exist('rtidc'), try,  rtidc('DataHostBlockClbNameChange', gcbh); catch, disp(['Warning: ''NameChangeFcn'' for RTI Data block failed: ' lasterr]); end, end,"
      mask Help:
      | RTI Data Block.
      | This block is used by RTI to store internal model-dependent data.
      | Please keep this block on the root level of the model. Deleting this block will result in data loss.
      | 
      | NEVER DELETE OR COPY THIS BLOCK!
      mask Display:
      | text(0.5, 0.5, 'RTI Data', 'HorizontalAlignment', 'center');
      | plot([1 0]);
  Sum : Sum  Inputs=|++
  Sum1 : Sum  Inputs=|++
  Switch1 : Switch  Threshold=1
  Switch2 : Switch  Threshold=1
  Tracking Force [N] : Constant  Value=5
  Tracking Force [N]1 : Constant  Value=5
  Tracking Subsys : Subsystem
  Tracking Subsys1 : Subsystem
  "pert_time 1 [ms] " : Constant  Value=100
  "pert_time 2 [ms] " : Constant  Value=100
  "zero offset " : Constant  Value=0
  zero offset 1 : Constant  Value=0
  wires:
  Constant1/1 -> Enabled Delay/1
  Enabled Delay/1 -> Switch1/2
  "Motor 1 On "/1 -> Motor Direction1/1
  Force Sensor Input [V]1/1 -> Analog Filter Design1/1
  Force Sensor Conversion [N/V] 1/1 -> F_meas [N]1/1
  "Perturbation 1 "/1 -> Enabled Delay/4, Enabled Delay/3
  Force Desired 1 [N]/1 -> Pertubration Subsys/1(In1)
  Pertubration Subsys/1(Out1) -> Switch1/1
  Tracking Force [N]/1 -> Tracking Subsys/1(In1)
  Tracking Subsys/1(Out1) -> Switch1/3
  Constant2/1 -> Product1/1
  Switch1/1 -> Product1/2
  Product1/1 -> Motor Command/1
  Analog Filter Design1/1 -> F_meas [N]1/2
  "zero offset "/1 -> Sum/2
  F_meas [N]1/1 -> Sum/1
  Sum/1 -> Tracking Subsys/2(In2), Pertubration Subsys/2(In2)
  "pert_time 1 [ms] "/1 -> Enabled Delay/2
  Tracking Force [N]1/1 -> Tracking Subsys1/1(In1)
  Constant3/1 -> Enabled Delay1/1
  Sum1/1 -> Tracking Subsys1/2(In2), Pertubration Subsys1/2(In2)
  "pert_time 2 [ms] "/1 -> Enabled Delay1/2
  F_meas [N]2/1 -> Sum1/1
  Constant4/1 -> Product2/1
  Switch2/1 -> Product2/2
  Force Sensor Input [V]2/1 -> Analog Filter Design2/1
  Enabled Delay1/1 -> Switch2/2
  Perturbation 2/1 -> Enabled Delay1/4, Enabled Delay1/3
  Force Sensor Conversion [N/V] 2/1 -> F_meas [N]2/1
  Product2/1 -> Motor Command1/1
  Pertubration Subsys1/1(Out1) -> Switch2/1
  Analog Filter Design2/1 -> F_meas [N]2/2
  "Motor 2 On "/1 -> Motor Direction2/1
  zero offset 1/1 -> Sum1/2
  Tracking Subsys1/1(Out1) -> Switch2/3
  "Force Desired 2 [N] "/1 -> Pertubration Subsys1/1(In1)

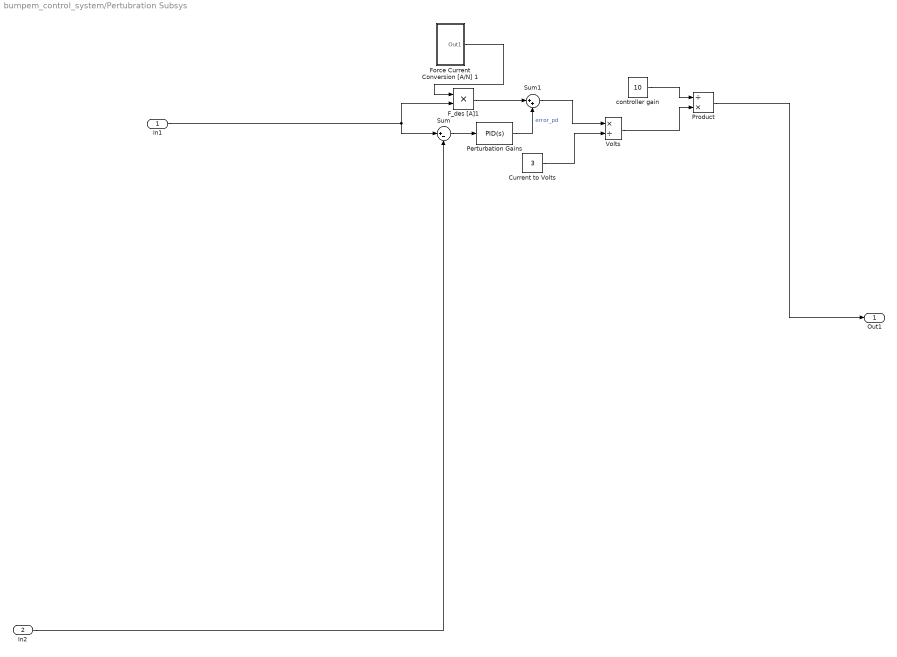
== system bumpem_control_system/Pertubration Subsys ==
  In1 : Inport
  In2 : Inport  Port=2
  "Current to Volts " : Constant  Value=3
  F_des [A]1 : Product
  Force Current Conversion [A/N] 1 : Subsystem
  Perturbation Gains : simulink/Continuous/PID Controller  Controller=PID  TimeDomain=Continuous-time  SampleTime=-1  IntegratorMethod=Forward Euler  FilterMethod=Forward Euler  Form=Parallel  UseFilter=on  ControllerParametersSource=internal  P=.000001  I=0  D=.0016  N=100  InitialConditionSource=internal  InitialConditionForIntegrator=0  InitialConditionForFilter=0  ExternalReset=none  LimitOutput=off  UpperSaturationLimit=inf  LowerSaturationLimit=-inf  LinearizeAsGain=on  AntiWindupMode=none  Kb=1  TrackingMode=off  Kt=1  PParamMin=[]  PParamMax=[]  IParamMin=[]  IParamMax=[]  DParamMin=[]  DParamMax=[]  NParamMin=[]  NParamMax=[]  KbParamMin=[]  KbParamMax=[]  KtParamMin=[]  KtParamMax=[]  POutMin=[]  POutMax=[]  IOutMin=[]  IOutMax=[]  DOutMin=[]  DOutMax=[]  NOutMin=[]  NOutMax=[]  KbOutMin=[]  KbOutMax=[]  KtOutMin=[]  KtOutMax=[]  IntegratorOutMin=[]  IntegratorOutMax=[]  FilterOutMin=[]  FilterOutMax=[]  SumOutMin=[]  SumOutMax=[]  SumI1OutMin=[]  SumI1OutMax=[]  SumI2OutMin=[]  SumI2OutMax=[]  SumI3OutMin=[]  SumI3OutMax=[]  SumDOutMin=[]  SumDOutMax=[]  SaturationOutMin=[]  SaturationOutMax=[]  IntegratorContinuousStateAttributes=''  IntegratorStateMustResolveToSignalObject=off  IntegratorRTWStateStorageClass=Auto  FilterContinuousStateAttributes=''  FilterStateMustResolveToSignalObject=off  FilterRTWStateStorageClass=Auto  DifferentiatorICPrevScaledInput=0  DifferentiatorOutMin=[]  DifferentiatorOutMax=[]  FilterDiffOutCoefMin=[]  FilterDiffOutCoefMax=[]  SumDenOutMin=[]  SumDenOutMax=[]  SumNumOutMin=[]  SumNumOutMax=[]  ReciprocalOutMin=[]  ReciprocalOutMax=[]  DivideOutMin=[]  DivideOutMax=[]  TunerSelectOption=Transfer Function Based (PID Tuner App)
  Product : Product  Inputs=/*
  Sum : Sum  Inputs=|+-
  Sum1 : Sum  Inputs=|++
  Volts : Product  Inputs=*/
  controller gain : Constant  Value=10
  Out1 : Outport
  wires:
  Sum/1 -> Perturbation Gains/1
  controller gain/1 -> Product/1
  Sum1/1 -> Volts/1
  "Current to Volts "/1 -> Volts/2
  In1/1 -> F_des [A]1/2, Sum/1
  Perturbation Gains/1 -> Sum1/2  "error_pd"
  Volts/1 -> Product/2
  Product/1 -> Out1/1
  In2/1 -> Sum/2
  F_des [A]1/1 -> Sum1/1
  Force Current Conversion [A/N] 1/1(Out1) -> F_des [A]1/1

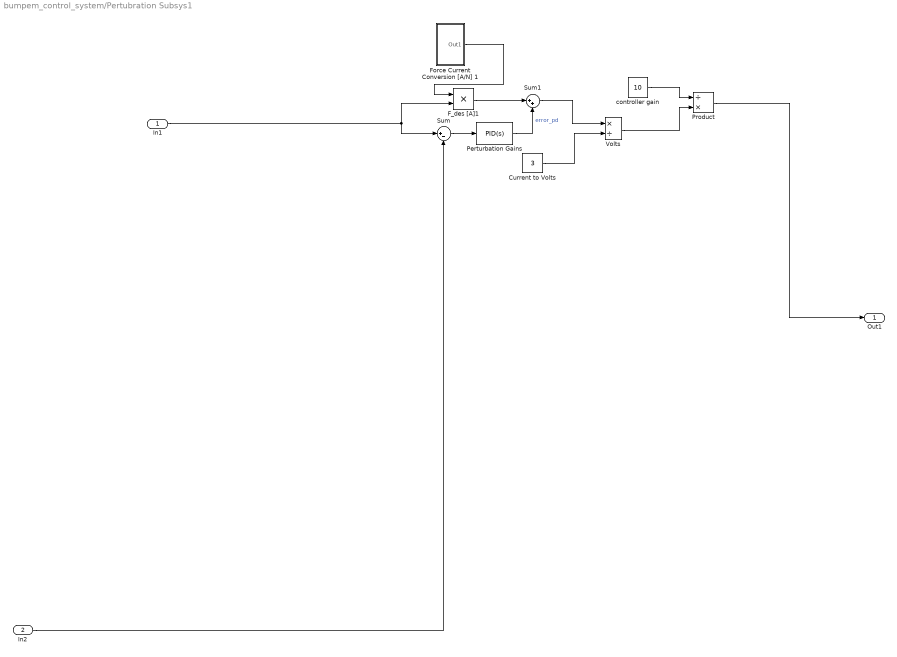
== system bumpem_control_system/Pertubration Subsys1 ==
  In1 : Inport
  In2 : Inport  Port=2
  "Current to Volts " : Constant  Value=3
  F_des [A]1 : Product
  Force Current Conversion [A/N] 1 : Subsystem
  Perturbation Gains : simulink/Continuous/PID Controller  Controller=PID  TimeDomain=Continuous-time  SampleTime=-1  IntegratorMethod=Forward Euler  FilterMethod=Forward Euler  Form=Parallel  UseFilter=on  ControllerParametersSource=internal  P=.000001  I=0  D=.0016  N=100  InitialConditionSource=internal  InitialConditionForIntegrator=0  InitialConditionForFilter=0  ExternalReset=none  LimitOutput=off  UpperSaturationLimit=inf  LowerSaturationLimit=-inf  LinearizeAsGain=on  AntiWindupMode=none  Kb=1  TrackingMode=off  Kt=1  PParamMin=[]  PParamMax=[]  IParamMin=[]  IParamMax=[]  DParamMin=[]  DParamMax=[]  NParamMin=[]  NParamMax=[]  KbParamMin=[]  KbParamMax=[]  KtParamMin=[]  KtParamMax=[]  POutMin=[]  POutMax=[]  IOutMin=[]  IOutMax=[]  DOutMin=[]  DOutMax=[]  NOutMin=[]  NOutMax=[]  KbOutMin=[]  KbOutMax=[]  KtOutMin=[]  KtOutMax=[]  IntegratorOutMin=[]  IntegratorOutMax=[]  FilterOutMin=[]  FilterOutMax=[]  SumOutMin=[]  SumOutMax=[]  SumI1OutMin=[]  SumI1OutMax=[]  SumI2OutMin=[]  SumI2OutMax=[]  SumI3OutMin=[]  SumI3OutMax=[]  SumDOutMin=[]  SumDOutMax=[]  SaturationOutMin=[]  SaturationOutMax=[]  IntegratorContinuousStateAttributes=''  IntegratorStateMustResolveToSignalObject=off  IntegratorRTWStateStorageClass=Auto  FilterContinuousStateAttributes=''  FilterStateMustResolveToSignalObject=off  FilterRTWStateStorageClass=Auto  DifferentiatorICPrevScaledInput=0  DifferentiatorOutMin=[]  DifferentiatorOutMax=[]  FilterDiffOutCoefMin=[]  FilterDiffOutCoefMax=[]  SumDenOutMin=[]  SumDenOutMax=[]  SumNumOutMin=[]  SumNumOutMax=[]  ReciprocalOutMin=[]  ReciprocalOutMax=[]  DivideOutMin=[]  DivideOutMax=[]  TunerSelectOption=Transfer Function Based (PID Tuner App)
  Product : Product  Inputs=/*
  Sum : Sum  Inputs=|+-
  Sum1 : Sum  Inputs=|++
  Volts : Product  Inputs=*/
  controller gain : Constant  Value=10
  Out1 : Outport
  wires:
  Sum/1 -> Perturbation Gains/1
  controller gain/1 -> Product/1
  Sum1/1 -> Volts/1
  "Current to Volts "/1 -> Volts/2
  In1/1 -> F_des [A]1/2, Sum/1
  Perturbation Gains/1 -> Sum1/2  "error_pd"
  Volts/1 -> Product/2
  Product/1 -> Out1/1
  In2/1 -> Sum/2
  F_des [A]1/1 -> Sum1/1
  Force Current Conversion [A/N] 1/1(Out1) -> F_des [A]1/1

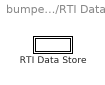
== system bumpem_control_system/RTI Data ==
  RTI Data Store : Subsystem  Tag="struct('private',struct('version',struct('dsVer',uint32(2),'dsVerCreation',uint32(2),'RTI',struct('ver','7.10','type','RTI1202')),'access',struct('type','Model','isPerm',1,'created',['13-Dec-2022 00:26:21'],'modified',['14-Feb-2023 21:14:22'],'location','')),'public',struct('main',struct('data',[]),'sub',struct('name',{{'latest_version_control_system_v2'}},'data',{{struct('TH',struct('thTaskInfo',struct('taskType',{'TIMER','HWINT','TMRINT','SWINT','GLINT'},'tasksNumOf',{1,0,0,0,0},'srcIds',{{'TIMERA'},{},{},{},{}},'taskNames',{{['Timer Task 1']},{},{},{},{}})),'th_tc',struct('dataType','TASK','taskGroupId','','taskGroupList',{{}},'taskSchedulingPolicy','FCFS','taskType','TIMER','blkh',-1,'srcId','TIMERA','srcSgnName',['Timer A interrupt'],'srcCpuName','','taskName',['Timer Task 1  [0.001] s'],'taskNameDisplayExt','','smplTime',0.001,'smplTimeOffs',0,'hasFixedPriority',0,'priority',1,'hasFixedOvc',0,'ovcType',1,'ovcMax',1),'tc_th',struct('dataType','TASK','taskGroupId','','taskGroupList',{{}},'taskSchedulingPolicy','FCFS','taskType','TIMER','blkh',-1,'srcId','TIMERA','srcSgnName',['Timer A interrupt'],'srcCpuName','','taskName',['Timer Task 1  [0.001] s'],'taskNameDisplayExt','','smplTime',0.001,'smplTimeOffs',0,'hasFixedPriority',0,'priority',1,'hasFixedOvc',0,'ovcType',1,'ovcMax',1))}})))"  mask(RTI_DATA_STORE){}
      mask help:
      | RTI Data Store Block. This block is used by RTI to store internal model dependent data. Deleting this block will result in data loss.
      |
      | NEVER DELETE, COPY, OR MODIFY THIS BLOCK!
      mask Help:
      | RTI Data Store Block. This block is used by RTI to store internal model dependent data. Deleting this block will result in data loss.
      | 
      | NEVER DELETE, COPY, OR MODIFY THIS BLOCK!
      mask Display: text(0.5, 0.5, ' ', 'HorizontalAlignment', 'center');

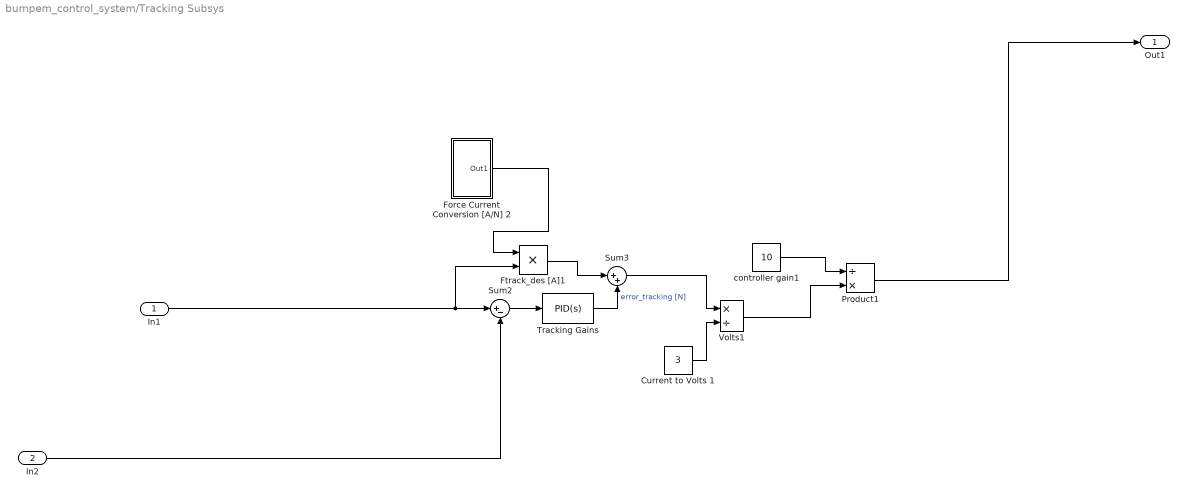
== system bumpem_control_system/Tracking Subsys ==
  In1 : Inport
  In2 : Inport  Port=2
  Current to Volts 1 : Constant  Value=3
  Force Current Conversion [A/N] 2 : Subsystem
  Ftrack_des [A]1 : Product
  Product1 : Product  Inputs=/*
  Sum2 : Sum  Inputs=|+-
  Sum3 : Sum  Inputs=|++
  Tracking Gains : simulink/Continuous/PID Controller  Controller=PID  TimeDomain=Continuous-time  SampleTime=-1  IntegratorMethod=Forward Euler  FilterMethod=Forward Euler  Form=Parallel  UseFilter=on  ControllerParametersSource=internal  P=0  I=0  D=0  N=100  InitialConditionSource=internal  InitialConditionForIntegrator=0  InitialConditionForFilter=0  ExternalReset=none  LimitOutput=off  UpperSaturationLimit=inf  LowerSaturationLimit=-inf  LinearizeAsGain=on  AntiWindupMode=none  Kb=1  TrackingMode=off  Kt=1  PParamMin=[]  PParamMax=[]  IParamMin=[]  IParamMax=[]  DParamMin=[]  DParamMax=[]  NParamMin=[]  NParamMax=[]  KbParamMin=[]  KbParamMax=[]  KtParamMin=[]  KtParamMax=[]  POutMin=[]  POutMax=[]  IOutMin=[]  IOutMax=[]  DOutMin=[]  DOutMax=[]  NOutMin=[]  NOutMax=[]  KbOutMin=[]  KbOutMax=[]  KtOutMin=[]  KtOutMax=[]  IntegratorOutMin=[]  IntegratorOutMax=[]  FilterOutMin=[]  FilterOutMax=[]  SumOutMin=[]  SumOutMax=[]  SumI1OutMin=[]  SumI1OutMax=[]  SumI2OutMin=[]  SumI2OutMax=[]  SumI3OutMin=[]  SumI3OutMax=[]  SumDOutMin=[]  SumDOutMax=[]  SaturationOutMin=[]  SaturationOutMax=[]  IntegratorContinuousStateAttributes=''  IntegratorStateMustResolveToSignalObject=off  IntegratorRTWStateStorageClass=Auto  FilterContinuousStateAttributes=''  FilterStateMustResolveToSignalObject=off  FilterRTWStateStorageClass=Auto  DifferentiatorICPrevScaledInput=0  DifferentiatorOutMin=[]  DifferentiatorOutMax=[]  FilterDiffOutCoefMin=[]  FilterDiffOutCoefMax=[]  SumDenOutMin=[]  SumDenOutMax=[]  SumNumOutMin=[]  SumNumOutMax=[]  ReciprocalOutMin=[]  ReciprocalOutMax=[]  DivideOutMin=[]  DivideOutMax=[]  TunerSelectOption=Transfer Function Based (PID Tuner App)
  Volts1 : Product  Inputs=*/
  controller gain1 : Constant  Value=10
  Out1 : Outport
  wires:
  controller gain1/1 -> Product1/1
  Tracking Gains/1 -> Sum3/2  "error_tracking [N]"
  Current to Volts 1/1 -> Volts1/2
  In1/1 -> Ftrack_des [A]1/2, Sum2/1
  Volts1/1 -> Product1/2
  Sum3/1 -> Volts1/1
  Sum2/1 -> Tracking Gains/1
  Product1/1 -> Out1/1
  In2/1 -> Sum2/2
  Ftrack_des [A]1/1 -> Sum3/1
  Force Current Conversion [A/N] 2/1(Out1) -> Ftrack_des [A]1/1

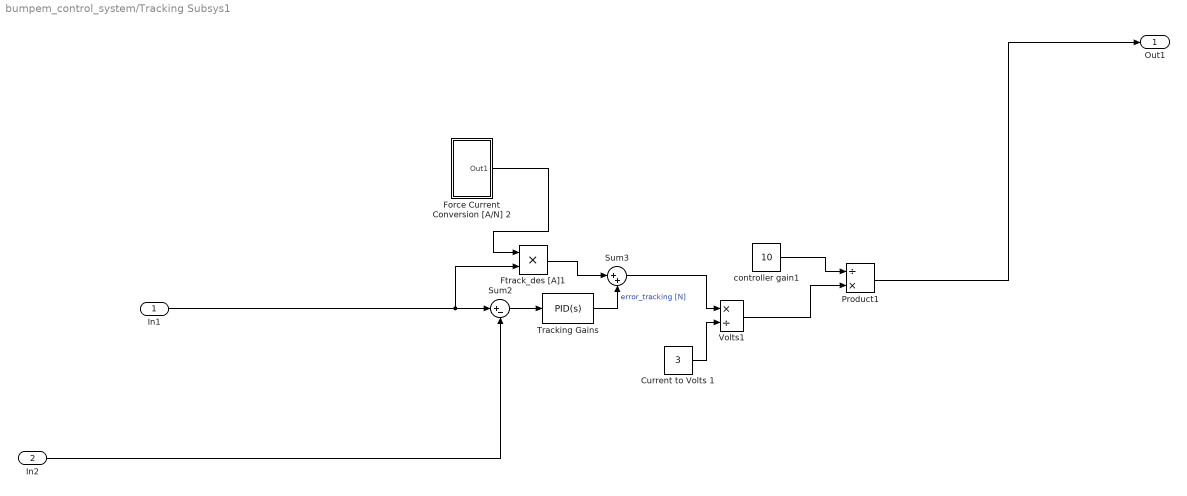
== system bumpem_control_system/Tracking Subsys1 ==
  In1 : Inport
  In2 : Inport  Port=2
  Current to Volts 1 : Constant  Value=3
  Force Current Conversion [A/N] 2 : Subsystem
  Ftrack_des [A]1 : Product
  Product1 : Product  Inputs=/*
  Sum2 : Sum  Inputs=|+-
  Sum3 : Sum  Inputs=|++
  Tracking Gains : simulink/Continuous/PID Controller  Controller=PID  TimeDomain=Continuous-time  SampleTime=-1  IntegratorMethod=Forward Euler  FilterMethod=Forward Euler  Form=Parallel  UseFilter=on  ControllerParametersSource=internal  P=0  I=0  D=0  N=100  InitialConditionSource=internal  InitialConditionForIntegrator=0  InitialConditionForFilter=0  ExternalReset=none  LimitOutput=off  UpperSaturationLimit=inf  LowerSaturationLimit=-inf  LinearizeAsGain=on  AntiWindupMode=none  Kb=1  TrackingMode=off  Kt=1  PParamMin=[]  PParamMax=[]  IParamMin=[]  IParamMax=[]  DParamMin=[]  DParamMax=[]  NParamMin=[]  NParamMax=[]  KbParamMin=[]  KbParamMax=[]  KtParamMin=[]  KtParamMax=[]  POutMin=[]  POutMax=[]  IOutMin=[]  IOutMax=[]  DOutMin=[]  DOutMax=[]  NOutMin=[]  NOutMax=[]  KbOutMin=[]  KbOutMax=[]  KtOutMin=[]  KtOutMax=[]  IntegratorOutMin=[]  IntegratorOutMax=[]  FilterOutMin=[]  FilterOutMax=[]  SumOutMin=[]  SumOutMax=[]  SumI1OutMin=[]  SumI1OutMax=[]  SumI2OutMin=[]  SumI2OutMax=[]  SumI3OutMin=[]  SumI3OutMax=[]  SumDOutMin=[]  SumDOutMax=[]  SaturationOutMin=[]  SaturationOutMax=[]  IntegratorContinuousStateAttributes=''  IntegratorStateMustResolveToSignalObject=off  IntegratorRTWStateStorageClass=Auto  FilterContinuousStateAttributes=''  FilterStateMustResolveToSignalObject=off  FilterRTWStateStorageClass=Auto  DifferentiatorICPrevScaledInput=0  DifferentiatorOutMin=[]  DifferentiatorOutMax=[]  FilterDiffOutCoefMin=[]  FilterDiffOutCoefMax=[]  SumDenOutMin=[]  SumDenOutMax=[]  SumNumOutMin=[]  SumNumOutMax=[]  ReciprocalOutMin=[]  ReciprocalOutMax=[]  DivideOutMin=[]  DivideOutMax=[]  TunerSelectOption=Transfer Function Based (PID Tuner App)
  Volts1 : Product  Inputs=*/
  controller gain1 : Constant  Value=10
  Out1 : Outport
  wires:
  controller gain1/1 -> Product1/1
  Tracking Gains/1 -> Sum3/2  "error_tracking [N]"
  Current to Volts 1/1 -> Volts1/2
  In1/1 -> Ftrack_des [A]1/2, Sum2/1
  Volts1/1 -> Product1/2
  Sum3/1 -> Volts1/1
  Sum2/1 -> Tracking Gains/1
  Product1/1 -> Out1/1
  In2/1 -> Sum2/2
  Ftrack_des [A]1/1 -> Sum3/1
  Force Current Conversion [A/N] 2/1(Out1) -> Ftrack_des [A]1/1
